simulink model "slrt_udp"  (R2023a)
settings: Solver=FixedStepDiscrete  StartTime=0.0  StopTime=Inf  RelTol=1e-3  EnableMultiTasking=on
model workspace (MAT data in the model file):
  upd_size = 16384
libraries: slrealtimeiplib x1
settings Model: SimulationMode=external  ExtModeEnableFloating=off  ParameterArgumentNames=upd_size  Creator=The MathWorks, Inc.  LastModifiedBy=sr810
settings SolverCC: ConcurrentTasks=on  AlgebraicLoopSolver=TrustRegion  PositivePriorityOrder=on  InsertRTBMode=Never (minimum delay)  MaxZcPerStep=1
settings DataIOCC: SaveFormat=Array  SaveState=on  SignalLoggingName=logsOut
settings OptimizationCC: BlockReduction=off  BooleanDataType=off  OptimizeBlockIOStorage=off  BufferReuse=off  GlobalBufferReuse=off  ExpressionFolding=off  LocalBlockOutputs=off  InitFltsAndDblsToZero=on  OptimizeDataStoreBuffers=off  BusAssignmentInplaceUpdate=off
settings DebuggingCC: SaveWithParameterizedLinksMsg=none  UnderspecifiedInitializationDetection=Classic  MergeDetectMultiDrivingBlocksExec=none  CheckExecutionContextPreStartOutputMsg=on  SignalResolutionControl=TryResolveAllWithWarning  TasksWithSamePriorityMsg=none  UnconnectedInputMsg=warning  UnconnectedOutputMsg=warning  UnconnectedLineMsg=warning  SFUnexpectedBacktrackingDiag=warning  SFNoUnconditionalDefaultTransitionDiag=warning  SFExecutionAtInitializationDiag=none  ArithmeticOperatorsInVariantConditions=warning
settings HardwareCC: ProdBitPerLong=64  ProdLongLongMode=on  ProdHWDeviceType=Intel->x86-64 (Linux 64)
settings ModelReferenceCC: EnableRefExpFcnMdlSchedulingChecks=on  PropagateSignalLabelsOutOfModel=off
settings SFSimCC: SimUseLocalCustomCode=off  SimTargetLang=C++
settings RTWCC: Description=Simulink Real-Time  SystemTargetFile=slrealtime.tlc  TemplateMakefile=slrealtime_default_tmf  RTWUseLocalCustomCode=off  Toolchain=Simulink Real-Time Toolchain  BuildConfiguration=Faster Runs  CodeExecutionProfiling=on  TargetLang=C++  DLArmComputeVersion=19.05
settings CodeAppCC: StateflowObjectComments=on
settings SimulinkRealTimeTargetCC: MATLABClassNameForMDSCustomization=Simulink.SoftwareTarget.GRTCustomization  UseGCCFastMath=on
settings ConfigComp: CovMetricSettings=dw  CovSaveCumulativeToWorkspaceVar=on  CovSaveSingleToWorkspaceVar=on  CovExternalEMLEnable=off  CovSFcnEnable=off

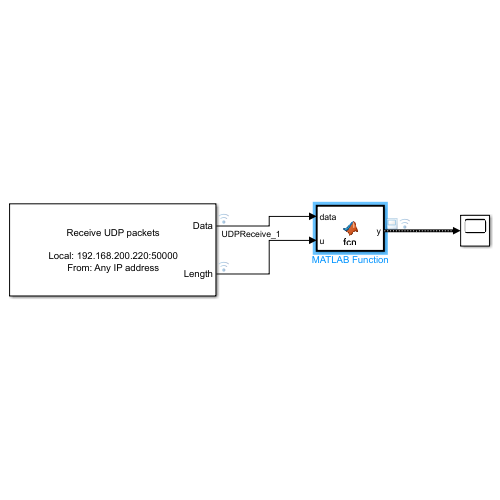
[thumbnail: Simulink's stored preview of the top-level diagram]
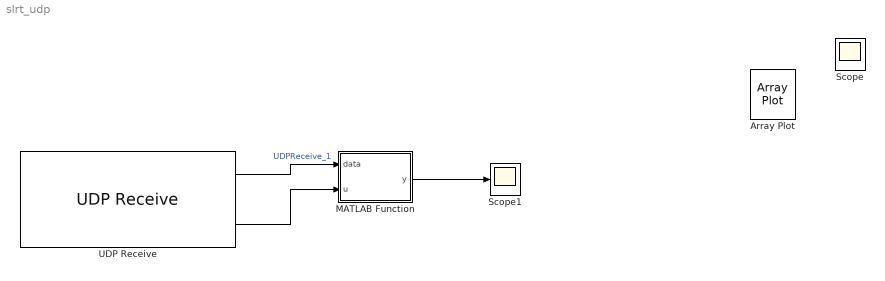
== system slrt_udp ==
  MATLAB Function : MATLAB Function  TreatAsAtomicUnit=on
  Scope1 : Scope
  UDP Receive : slrealtimeiplib/UDP Receive  useHostTargetConn=off  ipAddress=192.168.200.220  localPort=50000  rcvWidth=1228  rcvFmAny=on  fmAddress=192.168.200.200  sampleTime=0.01  enableMessage=off  maxPackets=1
  Array Plot : ArrayPlot  IOType=viewer  WindowPosition=[481.000000,141.000000,800.000000,500.000000,]  IsFloating=on  ScopeFrameLocation=window  PlotAsMagnitudePhase=on  YLimits=[0,10]  DefaultConfigurationName=dsp.scopes.ArrayPlotBlockSpecification
  Scope : Scope
  wires:
  UDP Receive/1 -> MATLAB Function/1(data)  "UDPReceive_1"
  UDP Receive/2 -> MATLAB Function/2(u)
  MATLAB Function/1(y) -> Scope1/1

== matlab function slrt_udp/MATLAB Function ==
  data: data input; u input; y output double size=20
function y  = fcn(data,u)
%tmp= read(app.rtEEG_obj.udpObj, app.rtEEG_obj.udpObj.NumBytesAvailable);
%[y]=rteeg_decode_bare(data(1:u));
%y=data(1);

numChannels=20;
numSampleBundles=20; %2000 Hz / 100 Hz
y=zeros(numChannels*numSampleBundles,1);

sample=uint8(data(29:28+3*numChannels*numSampleBundles));

rsample=reshape(sample,[3, length(sample)/3]);
rsample24=rteeg_read_int24(rsample);

y=reshape(rsample24, [numChannels, numSampleBundles]);
%y=randn(numChannels,1);
